simulink model "SimulinkSendReceive_multiple"  (R2024a)
settings: Solver=VariableStepAuto  StartTime=0.0  StopTime=15  RelTol=1e-3
undefined symbols (not defined in the file): LF
libraries: instrumentseriallib x3, svdutilitieslib x1
settings Model: Creator=Avell  LastModifiedBy=LENOVO
settings SolverCC: AlgebraicLoopSolver=TrustRegion
settings DataIOCC: ReturnWorkspaceOutputs=off
settings DebuggingCC: UnconnectedInputMsg=warning  UnconnectedOutputMsg=warning  UnconnectedLineMsg=warning  ArithmeticOperatorsInVariantConditions=warning
settings ModelReferenceCC: EnableRefExpFcnMdlSchedulingChecks=on
settings SFSimCC: SimUseLocalCustomCode=off  CustomCodeUndefinedFunction=UseInterfaceOnly
settings RTWCC: RTWUseLocalCustomCode=off  GPUComputeCapability=3.5

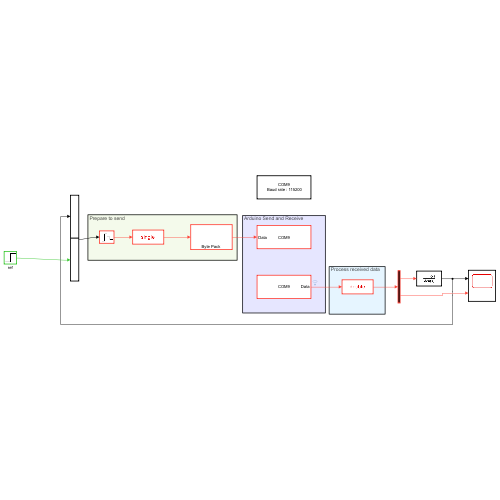
[thumbnail: Simulink's stored preview of the top-level diagram]
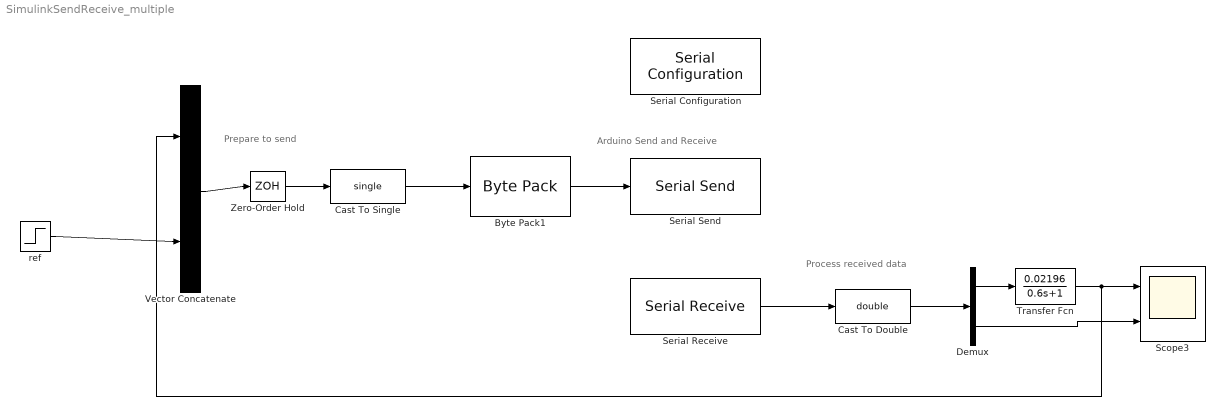
== system SimulinkSendReceive_multiple ==
  note: Process received data
  note: Prepare to send
  note: Arduino Send and Receive
  Byte Pack1 : svdutilitieslib/Byte Pack  maskPackedDataType=uint32  datatypes={'single'}  byteAlign=4  blockPlatform=arduinoert
  Cast To Double : DataTypeConversion  OutDataTypeStr=double  SaturateOnIntegerOverflow=off  RndMeth=Floor
  Cast To Single : DataTypeConversion  OutDataTypeStr=single  SaturateOnIntegerOverflow=off  RndMeth=Floor
  Demux : Demux  Outputs=2
  Scope3 : Scope  NumInputPorts=2
  Serial Configuration : instrumentseriallib/Serial Configuration  Priority=-200000  PortSel=COM9  Port=COM9  ComPort=COM9  BaudRate=115200  DataBits=8  Parity=none  StopBits=1  ByteOrder=little-endian  FlowControl=none  Timeout=10  SimulateUsing=Interpreted execution  BlockInModel=on  aMode=1
  Serial Receive : instrumentseriallib/Serial Receive  PortSel=COM9  Port=COM9  ComPort=COM9  DataType=single  SaveDataType=uint8  ToggleHeader=on  Header=[ 65 ]  ToggleDataSize=on  DataSize="[1  2]"  ToggleTerminator=on  Terminator=LF ('\n')  CustomTerminator=[]  InputFormat=Column major  EnableBlockingMode=on  ActionDataUnavailable=Output last received value  ActionWhenDataUnavailable=Output last received value  CustomValue=0  SampleTime=0.05  SimulateUsing=Interpreted execution  BlockInModel=on  aMode=1
  Serial Send : instrumentseriallib/Serial Send  PortSel=COM9  Port=COM9  ComPort=COM9  Header=[]  Terminator=<none>  CustomTerminator=[]  EnableBlockingMode=on  SimulateUsing=Interpreted execution  BlockInModel=on  aMode=1
  Transfer Fcn : TransferFcn  Numerator=[0.02196]  Denominator=[0.6 1]
  Vector Concatenate : Concatenate
  Zero-Order Hold : ZeroOrderHold  SampleTime=0.05
  ref : Step  SampleTime=0.1
  wires:
  Vector Concatenate/1 -> Zero-Order Hold/1
  Cast To Single/1 -> Byte Pack1/1
  Byte Pack1/1 -> Serial Send/1
  Serial Receive/1 -> Cast To Double/1
  Zero-Order Hold/1 -> Cast To Single/1
  Demux/2 -> Scope3/2
  Cast To Double/1 -> Demux/1
  Demux/1 -> Transfer Fcn/1
  Transfer Fcn/1 -> Scope3/1, Vector Concatenate/1
  ref/1 -> Vector Concatenate/2
